simulink model "dspilbc"  (Simulink 8.3)
settings: Solver=FixedStepDiscrete  StartTime=0.0  StopTime=inf  RelTol=1e-3
InitFcn:
  | ilbcDatatype = get_param([bdroot '/Configuration'],'ilbcDialogDatatype');
  | if strcmp(get_param([bdroot '/Configuration'],'ilbcDialogMode'), '13.33 kbit/sec mode')
  |   ilbcMode = 1;
  | else
  |   ilbcMode = 2;
  | end
model workspace: external: MAT-File dspilbcdata.mat (data not in the file)
undefined symbols (not defined in the file or in its folder): dfilt, ilbc, Newton, Raphson
libraries: simulink x36, dspmtrx3 x27, dspsigops x13, dsparch4 x10, dspquant2 x9, dspilbclib x8, dspstat3 x8, dspsrcs4 x2, dspvision x1, dspmisc x1, dspsnks4 x1, dsplp x1
(part 2 of 3)

== system dspilbc/iLBC Encoder/Create Packet (3.8)/Pack Packet ==
  Values : Inport
  Bitwise Operator1 : simulink/Logic and Bit Operations/Bitwise Operator  logicop=AND  UseBitMask=on  BitMask=128  BitMaskRealWorld=Stored Integer
  Bitwise Operator2 : simulink/Logic and Bit Operations/Bitwise Operator  logicop=AND  UseBitMask=on  BitMask=64  BitMaskRealWorld=Stored Integer
  Bitwise Operator3 : simulink/Logic and Bit Operations/Bitwise Operator  logicop=AND  UseBitMask=on  BitMask=32  BitMaskRealWorld=Stored Integer
  Bitwise Operator4 : simulink/Logic and Bit Operations/Bitwise Operator  logicop=AND  UseBitMask=on  BitMask=16  BitMaskRealWorld=Stored Integer
  Bitwise Operator5 : simulink/Logic and Bit Operations/Bitwise Operator  logicop=AND  UseBitMask=on  BitMask=8  BitMaskRealWorld=Stored Integer
  Bitwise Operator6 : simulink/Logic and Bit Operations/Bitwise Operator  logicop=AND  UseBitMask=on  BitMask=4  BitMaskRealWorld=Stored Integer
  Bitwise Operator7 : simulink/Logic and Bit Operations/Bitwise Operator  logicop=AND  UseBitMask=on  BitMask=2  BitMaskRealWorld=Stored Integer
  Bitwise Operator8 : simulink/Logic and Bit Operations/Bitwise Operator  logicop=AND  UseBitMask=on  BitMask=1  BitMaskRealWorld=Stored Integer
  Compare To Constant8 : simulink/Logic and Bit Operations/Compare To Constant  relop=~=  const=0  OutDataTypeStr=boolean  ZeroCross=off
  Constant : Constant  Value=[128 64 32 16 8 4 2 1]'  VectorParams1D=off  OutDataTypeStr=uint8
  Matrix Concatenate : Concatenate  NumInputs=8  Mode=Multidimensional array
  Matrix Multiply : Product  Multiplication=Matrix(*)  OutDataTypeStr=uint8
  Reshape : Reshape  OutputDimensionality=Customize  OutputDimensions=[ilbc.NO_OF_BYTES{ilbcMode} 8]
  Selector : Selector  NumberOfDimensions=2  InputPortWidth=3  IndexOptions=Index vector (dialog),Select all  Indices=ilbc.bit_packTbl{ilbcMode},1  OutputSizes=1,1
  Packet : Outport
  wires:
  Matrix Concatenate/1 -> Compare To Constant8/1
  Values/1 -> Bitwise Operator7/1, Bitwise Operator8/1, Bitwise Operator6/1, Bitwise Operator5/1, Bitwise Operator4/1, Bitwise Operator3/1, Bitwise Operator2/1, Bitwise Operator1/1
  Constant/1 -> Matrix Multiply/2
  Matrix Multiply/1 -> Packet/1
  Reshape/1 -> Matrix Multiply/1
  Selector/1 -> Reshape/1
  Bitwise Operator8/1 -> Matrix Concatenate/8
  Bitwise Operator7/1 -> Matrix Concatenate/7
  Bitwise Operator6/1 -> Matrix Concatenate/6
  Bitwise Operator5/1 -> Matrix Concatenate/5
  Bitwise Operator4/1 -> Matrix Concatenate/4
  Bitwise Operator3/1 -> Matrix Concatenate/3
  Bitwise Operator2/1 -> Matrix Concatenate/2
  Bitwise Operator1/1 -> Matrix Concatenate/1
  Compare To Constant8/1 -> Selector/1

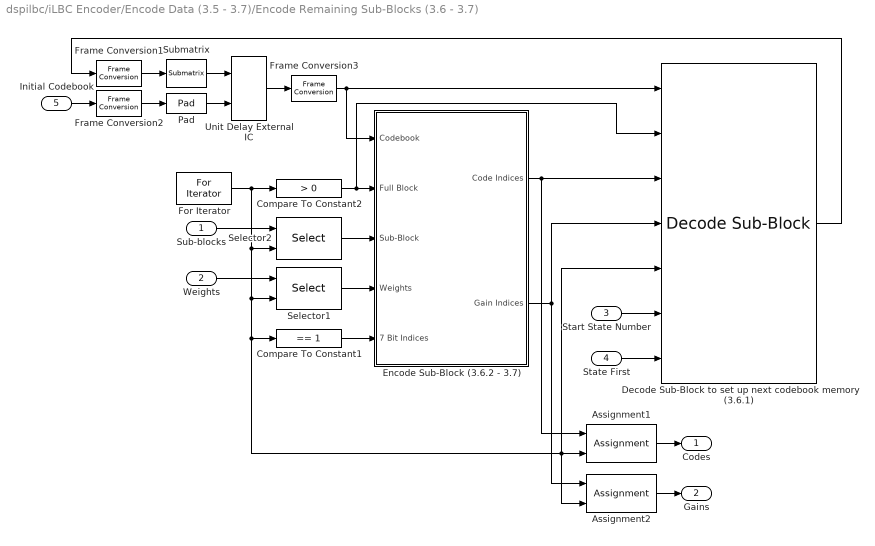
== system dspilbc/iLBC Encoder/Encode Data (3.5 - 3.7)/Encode Remaining Sub-Blocks (3.6 - 3.7) ==
  Sub-blocks : Inport
  Weights : Inport  Port=2
  Start State Number : Inport  Port=3
  State First : Inport  Port=4
  Initial Codebook : Inport  Port=5
  Assignment1 : Assignment  NumberOfDimensions=2  IndexMode=Zero-based  OutputInitialize=Specify size for each dimension in table  IndexOptions=Assign all,Index vector (port)  Indices=1,1  OutputSizes=3,ilbc.NSUB{ilbcMode}-1
  Assignment2 : Assignment  NumberOfDimensions=2  IndexMode=Zero-based  OutputInitialize=Specify size for each dimension in table  IndexOptions=Assign all,Index vector (port)  Indices=1,1  OutputSizes=3,ilbc.NSUB{ilbcMode}-1
  Compare To Constant1 : simulink/Logic and Bit Operations/Compare To Constant  relop===  const=1  OutDataTypeStr=uint8  ZeroCross=off
  Compare To Constant2 : simulink/Logic and Bit Operations/Compare To Constant  relop=>  const=0  OutDataTypeStr=uint8  ZeroCross=off
  Decode Sub-Block to set up next codebook memory (3.6.1) : dspilbclib/Decode Sub-Block
  Encode Sub-Block (3.6.2 - 3.7) : Subsystem  TreatAsAtomicUnit=on
  For Iterator : ForIterator  ResetStates=reset  IterationLimit=ilbc.NSUB{ilbcMode}-1  IndexMode=Zero-based
  Frame Conversion1 : FrameConversion  OutFrame=Sample-based
  Frame Conversion2 : FrameConversion  OutFrame=Sample-based
  Frame Conversion3 : FrameConversion
  Pad : dspsigops/Pad  padAlong=Columns  dimsToPad=1  valSrc=Specify via dialog  padVal=0  spec=Pad size  padNumOutRowsSpecMethod=User-specified  numOutRows=ilbc.BLOCKL{ilbcMode}-40  padNumOutColsSpecMethod=User-specified  numOutCols=1  isVarDimsMode=off  padBeginning=90  padEnd=0  outSizeMode=User-specified  outSize=1  padSigAt=Beginning  trunc_flag=None  roundingMode=Floor  overflowMode=off  truncOrWrapMode=Truncate  wrap_flag=None
  Selector1 : Selector  NumberOfDimensions=2  IndexMode=Zero-based  InputPortWidth=3  IndexOptions=Select all,Index vector (port)  Indices=-1,0
  Selector2 : Selector  NumberOfDimensions=2  IndexMode=Zero-based  InputPortWidth=3  IndexOptions=Select all,Index vector (port)  Indices=-1,0
  Submatrix : dspmtrx3/Submatrix  RowSpan=Range of rows  RowStartMode=Index  RowStartIndex=41  RowEndMode=Last  RowEndIndex=1  ColSpan=All columns  ColStartMode=First  ColStartIndex=1  ColEndMode=Last  ColEndIndex=1
  Unit Delay External IC : simulink/Additional Math & Discrete/Additional Discrete/Unit Delay External IC  tsamp=-1
  Codes : Outport
  Gains : Outport  Port=2
  wires:
  Encode Sub-Block (3.6.2 - 3.7)/2(Gain Indices) -> Assignment2/1, Decode Sub-Block to set up next codebook memory (3.6.1)/4
  Encode Sub-Block (3.6.2 - 3.7)/1(Code Indices) -> Assignment1/1, Decode Sub-Block to set up next codebook memory (3.6.1)/3
  Compare To Constant2/1 -> Encode Sub-Block (3.6.2 - 3.7)/2(Full Block), Decode Sub-Block to set up next codebook memory (3.6.1)/2
  Frame Conversion1/1 -> Submatrix/1
  Decode Sub-Block to set up next codebook memory (3.6.1)/1 -> Frame Conversion1/1
  Frame Conversion2/1 -> Pad/1
  For Iterator/1 -> Compare To Constant2/1, Selector2/2, Assignment2/2, Assignment1/2, Decode Sub-Block to set up next codebook memory (3.6.1)/5, Compare To Constant1/1, Selector1/2
  Frame Conversion3/1 -> Encode Sub-Block (3.6.2 - 3.7)/1(Codebook), Decode Sub-Block to set up next codebook memory (3.6.1)/1
  Assignment2/1 -> Gains/1
  Assignment1/1 -> Codes/1
  Weights/1 -> Selector1/1
  Sub-blocks/1 -> Selector2/1
  Initial Codebook/1 -> Frame Conversion2/1
  Compare To Constant1/1 -> Encode Sub-Block (3.6.2 - 3.7)/5(7 Bit Indices)
  Selector1/1 -> Encode Sub-Block (3.6.2 - 3.7)/4(Weights)
  Selector2/1 -> Encode Sub-Block (3.6.2 - 3.7)/3(Sub-Block)
  Submatrix/1 -> Unit Delay External IC/1
  Pad/1 -> Unit Delay External IC/2
  Unit Delay External IC/1 -> Frame Conversion3/1
  Start State Number/1 -> Decode Sub-Block to set up next codebook memory (3.6.1)/6
  State First/1 -> Decode Sub-Block to set up next codebook memory (3.6.1)/7

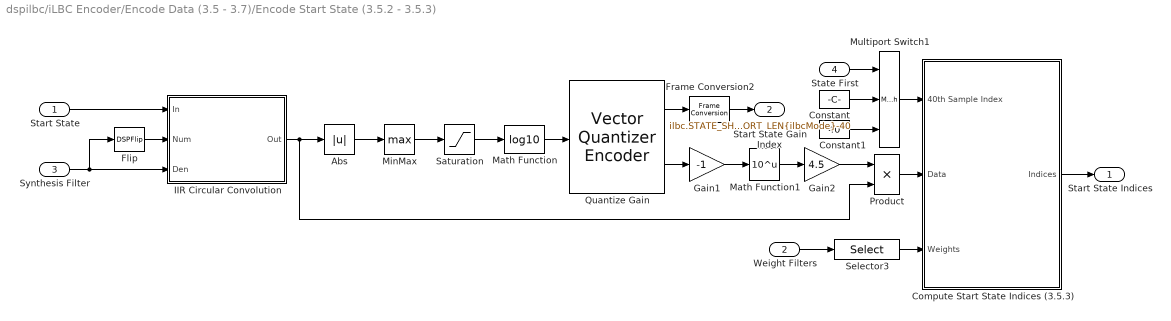
== system dspilbc/iLBC Encoder/Encode Data (3.5 - 3.7)/Encode Start State (3.5.2 - 3.5.3) ==
  Start State : Inport
  Weight Filters : Inport  Port=2
  Synthesis Filter : Inport  Port=3
  State First : Inport  Port=4
  Abs : Abs
  Compute Start State Indices (3.5.3) : Subsystem  TreatAsAtomicUnit=on
  Constant : Constant  Value=ilbc.STATE_SHORT_LEN{ilbcMode}-40  OutDataTypeStr=Inherit: Inherit via back propagation
  Constant1 : Constant  Value=40  OutDataTypeStr=Inherit: Inherit via back propagation
  Flip : DSPFlip
  Frame Conversion2 : FrameConversion  OutFrame=Sample-based
  Gain1 : Gain  Gain=-1  ParamDataTypeStr=Inherit: Same as input
  Gain2 : Gain  Gain=4.5  ParamDataTypeStr=Inherit: Same as input
  IIR Circular Convolution : Subsystem  TreatAsAtomicUnit=on
  Math Function : Math  Operator=log10  SaturateOnIntegerOverflow=on
  Math Function1 : Math  Operator=10^u  SaturateOnIntegerOverflow=on
  MinMax : MinMax  Function=max
  Multiport Switch1 : MultiPortSwitch  DataPortOrder=Zero-based contiguous  Inputs=2  zeroidx=on
  Product : Product  RndMeth=Zero
  Quantize Gain : dspquant2/Vector Quantizer Encoder  CBsource=Specify via dialog  codebook=ilbc.state_frgqTbl  distMeasure=Squared error  wgtSrc=Input port  weights=[1 1 1]  tieBreakRule=Choose the lower index  outQU=on  outQError=off  idtype=uint8  roundingMode=Floor  overflowMode=off
      settings: additionalParams=on
  Saturation : Saturate  UpperLimit=inf  LowerLimit=10
  Selector3 : Selector  NumberOfDimensions=2  InputPortWidth=3  IndexOptions=Index vector (dialog),Select all  Indices=2:11,-1
  Start State Indices : Outport
  Start State Gain Index : Outport  Port=2
  wires:
  Gain2/1 -> Product/1
  Product/1 -> Compute Start State Indices (3.5.3)/2(Data)
  Weight Filters/1 -> Selector3/1
  Multiport Switch1/1 -> Compute Start State Indices (3.5.3)/1(40th Sample Index)
  State First/1 -> Multiport Switch1/1
  Gain1/1 -> Math Function1/1
  IIR Circular Convolution/1(Out) -> Product/2, Abs/1
  Constant1/1 -> Multiport Switch1/3
  Constant/1 -> Multiport Switch1/2
  Selector3/1 -> Compute Start State Indices (3.5.3)/3(Weights)
  Math Function/1 -> Quantize Gain/1
  Math Function1/1 -> Gain2/1
  Frame Conversion2/1 -> Start State Gain Index/1
  Compute Start State Indices (3.5.3)/1(Indices) -> Start State Indices/1
  Start State/1 -> IIR Circular Convolution/1(In)
  Saturation/1 -> Math Function/1
  Synthesis Filter/1 -> IIR Circular Convolution/3(Den), Flip/1
  Quantize Gain/1 -> Frame Conversion2/1
  Quantize Gain/2 -> Gain1/1
  MinMax/1 -> Saturation/1
  Abs/1 -> MinMax/1
  Flip/1 -> IIR Circular Convolution/2(Num)

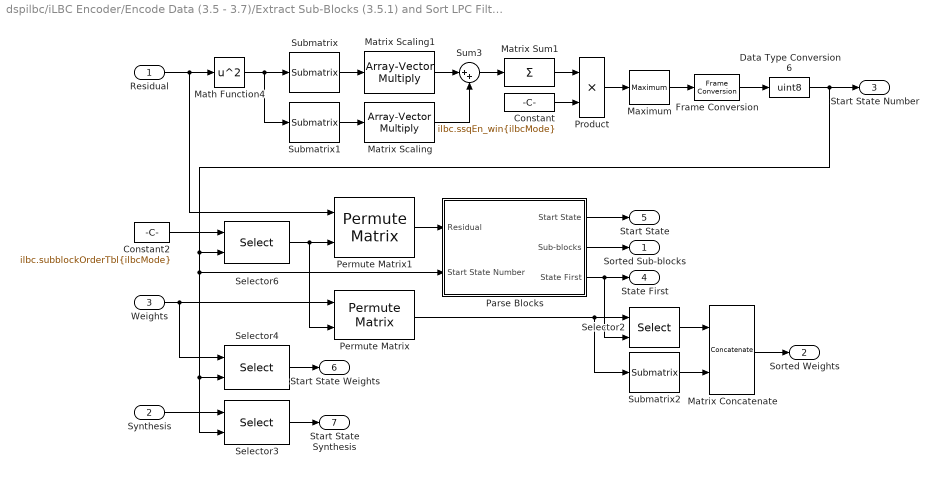
== system dspilbc/iLBC Encoder/Encode Data (3.5 - 3.7)/Extract Sub-Blocks (3.5.1) and Sort LPC Filters ==
  Residual : Inport
  Synthesis : Inport  Port=2
  Weights : Inport  Port=3
  Constant : Constant  Value=ilbc.ssqEn_win{ilbcMode}  VectorParams1D=off  OutDataTypeStr=Inherit: Inherit via back propagation
      settings: SamplingMode=Frame based
  Constant2 : Constant  Value=ilbc.subblockOrderTbl{ilbcMode}  OutDataTypeStr=uint8
  Data Type Conversion6 : DataTypeConversion  OutDataTypeStr=uint8
  Frame Conversion : FrameConversion  OutFrame=Sample-based
  Math Function4 : Math  Operator=square  SaturateOnIntegerOverflow=on
  Matrix Concatenate : Concatenate  Mode=Multidimensional array  ConcatenateDimension=2
  Matrix Scaling : dspmtrx3/Array-Vector Multiply  mode=Mute  saveAsFlag=0  Dimension=1  V_Source=Dialog parameter  V_VectFromMask=ilbc.sampEn_win2  firstCoeffSignedness=Auto  firstCoeffDataTypeStr=Inherit: Same word length as input  firstCoeffLastDataTypeStr=Inherit: Same word length as input  firstCoeffMin=[]  firstCoeffMax=[]  outputSignedness=Auto  outputMin=[]  outputMax=[]  accumSignedness=Auto  prodOutputSignedness=Auto  roundingMode=Floor  overflowMode=off
  Matrix Scaling1 : dspmtrx3/Array-Vector Multiply  mode=Mute  saveAsFlag=0  Dimension=1  V_Source=Dialog parameter  V_VectFromMask=ilbc.sampEn_win1  firstCoeffSignedness=Auto  firstCoeffDataTypeStr=Inherit: Same word length as input  firstCoeffLastDataTypeStr=Inherit: Same word length as input  firstCoeffMin=[]  firstCoeffMax=[]  outputSignedness=Auto  outputMin=[]  outputMax=[]  accumSignedness=Auto  prodOutputSignedness=Auto  roundingMode=Floor  overflowMode=off
  Matrix Sum1 : Sum  Inputs=+  CollapseMode=Specified dimension  OutDataTypeStr=Inherit: Same as accumulator
  Maximum : dspstat3/Maximum  fcn=Index  reset=None  InputProcessing=Columns as channels (frame based)  indexBase=One  operateOver=Each row  Dimension=1  colComp=on  operation=maximum  roiEnable=off  roiType=Rectangles  roiPortion=Entire ROI  roiOutput=Individual statistics for each ROI  roiFlag=off  accumDataTypeStr=Inherit: Same as product output  accumLastDataTypeStr=Inherit: Same as product output  roundingMode=Floor  overflowMode=off
  Parse Blocks : Subsystem
  Permute Matrix : dspmtrx3/Permute Matrix  mode=Columns  ZeroOneIdxMode=One-based  errmode=Clip index  checkDims=off
  Permute Matrix1 : dspmtrx3/Permute Matrix  mode=Columns  ZeroOneIdxMode=One-based  errmode=Clip index  checkDims=off
  Product : Product  RndMeth=Zero
  Selector2 : Selector  NumberOfDimensions=2  IndexMode=Zero-based  InputPortWidth=3  IndexOptions=Select all,Index vector (port)  Indices=-1,1:2
  Selector3 : Selector  NumberOfDimensions=2  InputPortWidth=3  IndexOptions=Select all,Index vector (port)  Indices=-1,-1  OutputSizes=2,2
  Selector4 : Selector  NumberOfDimensions=2  InputPortWidth=3  IndexOptions=Select all,Starting index (port)  Indices=-1,-1  OutputSizes=2,2
  Selector6 : Selector  NumberOfDimensions=2  InputPortWidth=3  IndexOptions=Index vector (port),Select all  Indices=-1,-1
  Submatrix : dspmtrx3/Submatrix  RowSpan=All rows  RowStartMode=First  RowStartIndex=1  RowEndMode=Last  RowEndIndex=1  ColSpan=Range of columns  ColStartMode=First  ColStartIndex=1  ColEndMode=Offset from last  ColEndIndex=1
  Submatrix1 : dspmtrx3/Submatrix  RowSpan=All rows  RowStartMode=First  RowStartIndex=1  RowEndMode=Last  RowEndIndex=1  ColSpan=Range of columns  ColStartMode=Index  ColStartIndex=2  ColEndMode=Last  ColEndIndex=1
  Submatrix2 : dspmtrx3/Submatrix  RowSpan=All rows  RowStartMode=Index  RowStartIndex=1  RowEndMode=Last  RowEndIndex=1  ColSpan=Range of columns  ColStartMode=Index  ColStartIndex=3  ColEndMode=Last  ColEndIndex=1
  Sum3 : Sum  Inputs=|++
  Sorted Sub-blocks : Outport
  Sorted Weights : Outport  Port=2
  Start State Number : Outport  Port=3
  State First : Outport  Port=4
  Start State : Outport  Port=5
  Start State Weights : Outport  Port=6
  Start State Synthesis : Outport  Port=7
  wires:
  Permute Matrix1/1 -> Parse Blocks/1(Residual)
  Selector6/1 -> Permute Matrix/2, Permute Matrix1/2
  Constant2/1 -> Selector6/1
  Data Type Conversion6/1 -> Selector6/2, Selector3/2, Selector4/2, Parse Blocks/2(Start State Number), Start State Number/1
  Matrix Concatenate/1 -> Sorted Weights/1
  Submatrix2/1 -> Matrix Concatenate/2
  Selector2/1 -> Matrix Concatenate/1
  Permute Matrix/1 -> Submatrix2/1, Selector2/1
  Selector4/1 -> Start State Weights/1
  Weights/1 -> Selector4/1, Permute Matrix/1
  Synthesis/1 -> Selector3/1
  Selector3/1 -> Start State Synthesis/1
  Frame Conversion/1 -> Data Type Conversion6/1
  Product/1 -> Maximum/1
  Constant/1 -> Product/2
  Matrix Sum1/1 -> Product/1
  Sum3/1 -> Matrix Sum1/1
  Matrix Scaling/1 -> Sum3/2
  Matrix Scaling1/1 -> Sum3/1
  Submatrix1/1 -> Matrix Scaling/1
  Submatrix/1 -> Matrix Scaling1/1
  Math Function4/1 -> Submatrix1/1, Submatrix/1
  Residual/1 -> Permute Matrix1/1, Math Function4/1
  Parse Blocks/2(Sub-blocks) -> Sorted Sub-blocks/1
  Parse Blocks/1(Start State) -> Start State/1
  Parse Blocks/3(State First) -> Selector2/2, State First/1
  Maximum/1 -> Frame Conversion/1

== system dspilbc/iLBC Encoder/Encoder LPC Analysis (3.2)/LSF Quantization (3.2.4) ==
  LSF Vectors : Inport
  Concatenation of Quantized LSFs : Concatenate  NumInputs=3  Mode=Multidimensional array
  Concatenation of Quantized LSFs1 : Concatenate  NumInputs=3  Mode=Multidimensional array
  Frame Conversion1 : FrameConversion  OutFrame=Sample-based
  Reshape : Reshape  OutputDimensionality=Column vector (2-D)
  Saturation : Saturate  UpperLimit=3.14  LowerLimit=0.01
  Selector1 : Selector  NumberOfDimensions=2  InputPortWidth=3  IndexOptions=Index vector (dialog),Select all  Indices=1:3,-1
  Selector2 : Selector  NumberOfDimensions=2  InputPortWidth=3  IndexOptions=Index vector (dialog),Select all  Indices=4:6,-1
  Selector3 : Selector  NumberOfDimensions=2  InputPortWidth=3  IndexOptions=Index vector (dialog),Select all  Indices=7:10,-1
  Sort : dspstat3/Sort  otype=Value  dir=Ascending  sortAlg=Quick sort  roundingMode=Floor  overflowMode=off
  VQ of LSF: 1st subvector : dspquant2/Vector Quantizer Encoder  CBsource=Specify via dialog  codebook=ilbc.lsfCbTbl1  distMeasure=Squared error  wgtSrc=Input port  weights=[1 1 1]  tieBreakRule=Choose the lower index  outQU=on  outQError=off  idtype=uint8  roundingMode=Floor  overflowMode=off
      settings: additionalParams=on
  VQ of LSF: 2nd subvector : dspquant2/Vector Quantizer Encoder  CBsource=Specify via dialog  codebook=ilbc.lsfCbTbl2  distMeasure=Squared error  wgtSrc=Input port  weights=[1 1 1]  tieBreakRule=Choose the lower index  outQU=on  outQError=off  idtype=uint8  roundingMode=Floor  overflowMode=off
      settings: additionalParams=on
  VQ of LSF: 3rd subvector : dspquant2/Vector Quantizer Encoder  CBsource=Specify via dialog  codebook=ilbc.lsfCbTbl3  distMeasure=Squared error  wgtSrc=Input port  weights=[1 1 1]  tieBreakRule=Choose the lower index  outQU=on  outQError=off  idtype=uint8  roundingMode=Floor  overflowMode=off
      settings: additionalParams=on
  LSF Indices : Outport
  Quantized LSF Vectors : Outport  Port=2
  wires:
  Reshape/1 -> Frame Conversion1/1
  Selector3/1 -> VQ of LSF: 3rd subvector/1
  Selector2/1 -> VQ of LSF: 2nd subvector/1
  Selector1/1 -> VQ of LSF: 1st subvector/1
  Frame Conversion1/1 -> LSF Indices/1
  VQ of LSF: 3rd subvector/1 -> Concatenation of Quantized LSFs1/3
  VQ of LSF: 2nd subvector/1 -> Concatenation of Quantized LSFs1/2
  VQ of LSF: 1st subvector/1 -> Concatenation of Quantized LSFs1/1
  Concatenation of Quantized LSFs1/1 -> Reshape/1
  Saturation/1 -> Quantized LSF Vectors/1
  LSF Vectors/1 -> Selector2/1, Selector3/1, Selector1/1
  Sort/1 -> Saturation/1
  VQ of LSF: 3rd subvector/2 -> Concatenation of Quantized LSFs/3
  Concatenation of Quantized LSFs/1 -> Sort/1
  VQ of LSF: 2nd subvector/2 -> Concatenation of Quantized LSFs/2
  VQ of LSF: 1st subvector/2 -> Concatenation of Quantized LSFs/1

== system dspilbc/iLBC Encoder/Encode Data (3.5 - 3.7)/Encode Remaining Sub-Blocks (3.6 - 3.7)/Encode Sub-Block (3.6.2 - 3.7) ==
  Codebook : Inport
  Full Block : Inport  Port=2
  Sub-Block : Inport  Port=3
  Weights : Inport  Port=4
  7 Bit Indices : Inport  Port=5
  3 Stage Sub-Block Encoder (3.6.4) : Subsystem  TreatAsAtomicUnit=on
  Adjust First Gain Index (3.7) : Subsystem  TreatAsAtomicUnit=on
  Compute Codebooks (3.6.2 - 3.6.3) : Subsystem
  Code Indices : Outport
  Gain Indices : Outport  Port=2
  wires:
  Codebook/1 -> Compute Codebooks (3.6.2 - 3.6.3)/1(Codebook)
  3 Stage Sub-Block Encoder (3.6.4)/4(Quantized Gain) -> Adjust First Gain Index (3.7)/4(Quantized Gain)
  3 Stage Sub-Block Encoder (3.6.4)/3(Quantized Target) -> Adjust First Gain Index (3.7)/3(Quantized Target)
  3 Stage Sub-Block Encoder (3.6.4)/2(Gain Indices) -> Adjust First Gain Index (3.7)/2(Gain Indices)
  3 Stage Sub-Block Encoder (3.6.4)/1(Code Indices) -> Code Indices/1
  Adjust First Gain Index (3.7)/1(Adjusted Gain Indices) -> Gain Indices/1
  Sub-Block/1 -> Compute Codebooks (3.6.2 - 3.6.3)/2(Sub-Block)
  Weights/1 -> Compute Codebooks (3.6.2 - 3.6.3)/3(Weights)
  Compute Codebooks (3.6.2 - 3.6.3)/1(Target) -> 3 Stage Sub-Block Encoder (3.6.4)/1(Target), Adjust First Gain Index (3.7)/1(Target)
  Compute Codebooks (3.6.2 - 3.6.3)/2(Codebooks) -> 3 Stage Sub-Block Encoder (3.6.4)/2(Codebooks)
  Compute Codebooks (3.6.2 - 3.6.3)/3(Augmented) -> 3 Stage Sub-Block Encoder (3.6.4)/3(Augmented)
  Compute Codebooks (3.6.2 - 3.6.3)/4(Norms) -> 3 Stage Sub-Block Encoder (3.6.4)/4("Norms ")
  Full Block/1 -> Compute Codebooks (3.6.2 - 3.6.3)/4(Full Block), 3 Stage Sub-Block Encoder (3.6.4)/6(Full Block)
  7 Bit Indices/1 -> 3 Stage Sub-Block Encoder (3.6.4)/5(7 Bit Indices)

== system dspilbc/iLBC Encoder/Encode Data (3.5 - 3.7)/Encode Start State (3.5.2 - 3.5.3)/Compute Start State Indices (3.5.3) ==
  40th Sample Index : Inport
  Data : Inport  Port=2
  Weights : Inport  Port=3
  Assignment : Assignment  NumberOfDimensions=2  OutputInitialize=Specify size for each dimension in table  IndexOptions=Index vector (port),Assign all  Indices=1,-1  OutputSizes=ilbc.STATE_SHORT_LEN{ilbcMode},1
  Delay : dspsigops/Delay  dly_unit=Samples  delay=1  ic_detail=off  dif_ic_for_ch=off  dif_ic_for_dly=off  ic=0  reset_popup=None
  Delay1 : dspsigops/Delay  dly_unit=Samples  delay=1  ic_detail=off  dif_ic_for_ch=off  dif_ic_for_dly=off  ic=0  reset_popup=None
  Dot Product : DotProduct  InputSameDT=on  OutDataTypeStr=Inherit: Inherit via internal rule
  Dot Product1 : DotProduct  InputSameDT=on  OutDataTypeStr=Inherit: Inherit via internal rule
  For Iterator : ForIterator  ResetStates=reset  IterationLimit=ilbc.STATE_SHORT_LEN{ilbcMode}
  Frame Conversion1 : FrameConversion  OutFrame=Sample-based
  Relational Operator : RelationalOperator  Operator=>  OutDataTypeStr=uint(8)
  Selector1 : Selector  NumberOfDimensions=2  IndexMode=Zero-based  InputPortWidth=3  IndexOptions=Select all,Index vector (port)  Indices=-1,-1
  Selector2 : Selector  NumberOfDimensions=2  InputPortWidth=3  IndexOptions=Index vector (port),Select all  Indices=-1,-1
  Sum : Sum  Inputs=+|+  OutDataTypeStr=Inherit: Inherit via back propagation
  Sum1 : Sum  Inputs=+-|
  Sum2 : Sum  Inputs=|-+
  Tapped Delay : simulink/Discrete/Tapped Delay  vinit=0.0  samptime=-1  NumDelays=9  DelayOrder=Newest  includeCurrent=on
  Tapped Delay1 : simulink/Discrete/Tapped Delay  vinit=0.0  samptime=-1  NumDelays=9  DelayOrder=Newest  includeCurrent=on
  Vector Quantizer Encoder : dspquant2/Vector Quantizer Encoder  CBsource=Specify via dialog  codebook=ilbc.state_sq3Tbl  distMeasure=Squared error  wgtSrc=Specify via dialog  weights=[1 1 1]  tieBreakRule=Choose the lower index  outQU=on  outQError=off  idtype=uint8  roundingMode=Floor  overflowMode=on
      settings: additionalParams=on
  Indices : Outport
  wires:
  For Iterator/1 -> Assignment/2, Selector2/2, Relational Operator/1
  Dot Product1/1 -> Sum2/1
  Delay1/1 -> Dot Product1/1
  Selector2/1 -> Sum2/2
  Sum2/1 -> Sum/1, Tapped Delay1/1
  Tapped Delay1/1 -> Delay1/1
  Sum1/1 -> Tapped Delay/1
  Tapped Delay/1 -> Delay/1
  Delay/1 -> Dot Product/2
  Dot Product/1 -> Sum1/2, Sum/2
  Selector1/1 -> Dot Product1/2, Dot Product/1
  Relational Operator/1 -> Selector1/2
  Weights/1 -> Selector1/1
  Data/1 -> Frame Conversion1/1
  Vector Quantizer Encoder/2 -> Sum1/1
  Vector Quantizer Encoder/1 -> Assignment/1
  Sum/1 -> Vector Quantizer Encoder/1
  40th Sample Index/1 -> Relational Operator/2
  Assignment/1 -> Indices/1
  Frame Conversion1/1 -> Selector2/1

== system dspilbc/iLBC Encoder/Encode Data (3.5 - 3.7)/Encode Start State (3.5.2 - 3.5.3)/IIR Circular Convolution ==
  In : Inport
  Num : Inport  Port=2
  Den : Inport  Port=3
  Digital Filter : dsparch4/Digital Filter  TypePopup=IIR (poles & zeros)  IIRFiltStruct=Direct form II transposed  AllPoleFiltStruct=Direct form  FIRFiltStruct=Direct form  CoeffSource=Input port(s)  NumCoeffs=[1 2]  DenCoeffs=[1 0.1]  BiQuadCoeffs=[1 0.3 0.4 1 0.1 0.2]  LatticeCoeffs=[0.2 0.4]  denIgnore=on  FiltPerSampPopup=One filter per frame  IC=0  ICnum=0  ICden=0  roundingMode=Floor  overflowMode=off  ScaleValues=1  scaleValueFracLength=14  stageInFracLength=15  stageOutFracLength=15  FilterSource=Input port(s)  dfiltObjectName=dfilt.dffir([1 2 1])  InputProcessing=Columns as channels (frame based)
  For Iterator : ForIterator  ResetStates=reset  IterationLimit=2  ShowIterationPort=off
  Out : Outport
  wires:
  Den/1 -> Digital Filter/3
  Num/1 -> Digital Filter/2
  In/1 -> Digital Filter/1
  Digital Filter/1 -> Out/1

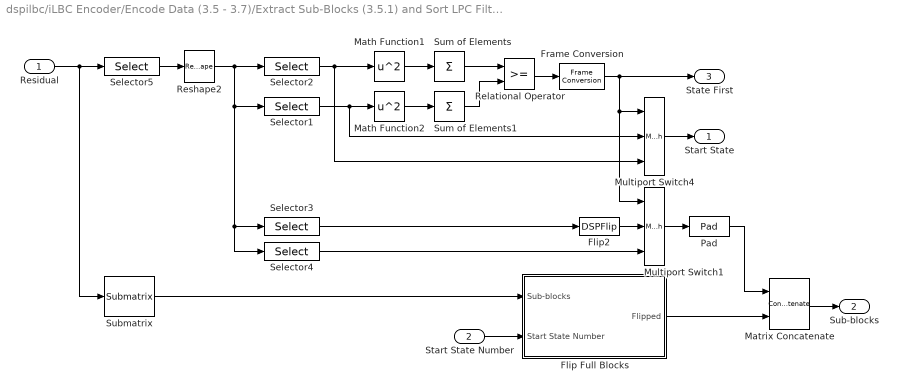
== system dspilbc/iLBC Encoder/Encode Data (3.5 - 3.7)/Extract Sub-Blocks (3.5.1) and Sort LPC Filters/Parse Blocks ==
  Residual : Inport
  Start State Number : Inport  Port=2
  Flip Full Blocks : Subsystem  TreatAsAtomicUnit=on
  Flip2 : DSPFlip
  Frame Conversion : FrameConversion  OutFrame=Sample-based
  Math Function1 : Math  Operator=square  SaturateOnIntegerOverflow=on
  Math Function2 : Math  Operator=square  SaturateOnIntegerOverflow=on
  Matrix Concatenate : Concatenate  Mode=Multidimensional array  ConcatenateDimension=2
  Multiport Switch1 : MultiPortSwitch  DataPortOrder=Zero-based contiguous  Inputs=2  zeroidx=on
  Multiport Switch4 : MultiPortSwitch  DataPortOrder=Zero-based contiguous  Inputs=2  zeroidx=on
  Pad : dspsigops/Pad  padAlong=Columns  dimsToPad=1  valSrc=Specify via dialog  padVal=0  spec=Output size  padNumOutRowsSpecMethod=User-specified  numOutRows=40  padNumOutColsSpecMethod=User-specified  numOutCols=1  isVarDimsMode=off  padBeginning=0  padEnd=0  outSizeMode=User-specified  outSize=1  padSigAt=End  trunc_flag=None  roundingMode=Floor  overflowMode=off  truncOrWrapMode=Truncate  wrap_flag=None
  Relational Operator : RelationalOperator  OutDataTypeStr=uint(8)
  Reshape2 : Reshape  OutputDimensionality=Column vector (2-D)
  Selector1 : Selector  NumberOfDimensions=2  InputPortWidth=3  IndexOptions=Index vector (dialog),Select all  Indices=(80-ilbc.STATE_SHORT_LEN{ilbcMode}+1):80,-1
  Selector2 : Selector  NumberOfDimensions=2  InputPortWidth=3  IndexOptions=Index vector (dialog),Select all  Indices=1:ilbc.STATE_SHORT_LEN{ilbcMode},-1
  Selector3 : Selector  NumberOfDimensions=2  InputPortWidth=3  IndexOptions=Starting index (dialog),Select all  Indices=1,-1  OutputSizes=80-ilbc.STATE_SHORT_LEN{ilbcMode},1
  Selector4 : Selector  NumberOfDimensions=2  InputPortWidth=3  IndexOptions=Index vector (dialog),Select all  Indices=(ilbc.STATE_SHORT_LEN{ilbcMode}+1):80,-1
  Selector5 : Selector  NumberOfDimensions=2  InputPortWidth=3  IndexOptions=Select all,Index vector (dialog)  Indices=1:ilbc.STATE_SHORT_LEN{ilbcMode},1:2
  Submatrix : dspmtrx3/Submatrix  RowSpan=All rows  RowStartMode=First  RowStartIndex=1  RowEndMode=Last  RowEndIndex=1  ColSpan=Range of columns  ColStartMode=Index  ColStartIndex=3  ColEndMode=Last  ColEndIndex=1
  Sum of Elements : Sum  Inputs=+
  Sum of Elements1 : Sum  Inputs=+
  Start State : Outport
  Sub-blocks : Outport  Port=2
  State First : Outport  Port=3
  wires:
  Start State Number/1 -> Flip Full Blocks/2(Start State Number)
  Flip2/1 -> Multiport Switch1/2
  Flip Full Blocks/1(Flipped) -> Matrix Concatenate/2
  Submatrix/1 -> Flip Full Blocks/1(Sub-blocks)
  Matrix Concatenate/1 -> Sub-blocks/1
  Pad/1 -> Matrix Concatenate/1
  Multiport Switch1/1 -> Pad/1
  Reshape2/1 -> Selector3/1, Selector4/1, Selector1/1, Selector2/1
  Multiport Switch4/1 -> Start State/1
  Selector5/1 -> Reshape2/1
  Residual/1 -> Selector5/1, Submatrix/1
  Math Function2/1 -> Sum of Elements1/1
  Math Function1/1 -> Sum of Elements/1
  Sum of Elements1/1 -> Relational Operator/2
  Relational Operator/1 -> Frame Conversion/1
  Frame Conversion/1 -> State First/1, Multiport Switch1/1, Multiport Switch4/1
  Sum of Elements/1 -> Relational Operator/1
  Selector3/1 -> Flip2/1
  Selector4/1 -> Multiport Switch1/3
  Selector1/1 -> Math Function2/1, Multiport Switch4/2
  Selector2/1 -> Multiport Switch4/3, Math Function1/1

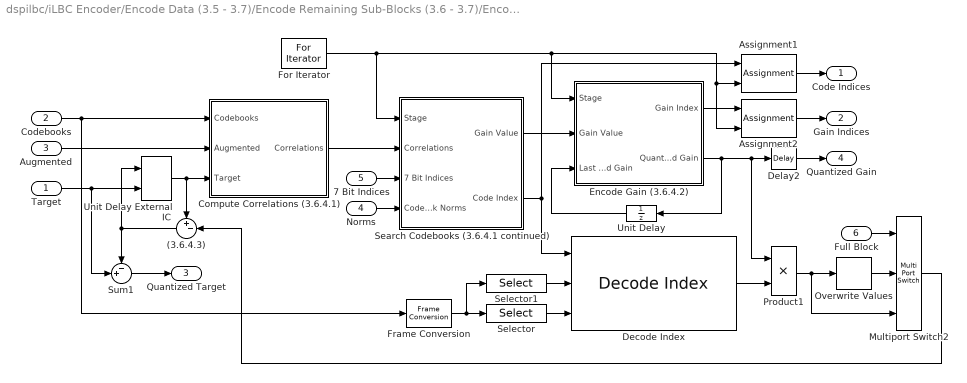
== system dspilbc/iLBC Encoder/Encode Data (3.5 - 3.7)/Encode Remaining Sub-Blocks (3.6 - 3.7)/Encode Sub-Block (3.6.2 - 3.7)/3 Stage Sub-Block Encoder (3.6.4) ==
  Target : Inport
  Codebooks : Inport  Port=2
  Augmented : Inport  Port=3
  "Norms " : Inport  Port=4
  7 Bit Indices : Inport  Port=5
  Full Block : Inport  Port=6
  (3.6.4.3) : Sum  Inputs=+-|
  Assignment1 : Assignment  NumberOfDimensions=2  IndexMode=Zero-based  OutputInitialize=Specify size for each dimension in table  IndexOptions=Index vector (port),Index vector (dialog)  Indices=1,0  OutputSizes=3,1
  Assignment2 : Assignment  NumberOfDimensions=2  IndexMode=Zero-based  OutputInitialize=Specify size for each dimension in table  IndexOptions=Index vector (port),Index vector (dialog)  Indices=1,0  OutputSizes=3,1
  Compute Correlations (3.6.4.1) : Subsystem  TreatAsAtomicUnit=on
  Decode Index : dspilbclib/Decode Index
  Delay2 : dspsigops/Delay  dly_unit=Samples  delay=2  ic_detail=off  dif_ic_for_ch=off  dif_ic_for_dly=off  ic=0  reset_popup=None
  Encode Gain (3.6.4.2) : Subsystem  TreatAsAtomicUnit=on
  For Iterator : ForIterator  ResetStates=reset  IterationLimit=3  IndexMode=Zero-based  IterationVariableDataType=int8
  Frame Conversion : FrameConversion  OutFrame=Sample-based
  Multiport Switch2 : MultiPortSwitch  DataPortOrder=Zero-based contiguous  Inputs=2  zeroidx=on
  Overwrite Values : dspmtrx3/Overwrite Values  OverWriteDiag=Submatrix  valFrom2ndIP=Specify via dialog  ConstValue=0  RowSpan=Range of rows  RowStartMode=First  RowStartIndex=1  RowEndMode=Offset from last  RowEndIndex=80-ilbc.STATE_SHORT_LEN{ilbcMode}  ColSpan=All columns  ColStartMode=First  ColStartIndex=1  ColEndMode=Last  ColEndIndex=1  DiagSpan=Range of elements  DiagStartMode=Index  DiagStartIndex=2  DiagEndMode=Index  DiagEndIndex=4
  Product1 : Product  RndMeth=Zero
  Search Codebooks (3.6.4.1 continued) : Subsystem  TreatAsAtomicUnit=on
  Selector : Selector  NumberOfDimensions=2  InputPortWidth=3  IndexOptions=Select all,Index vector (dialog)  Indices=[1 3],2  OutputSizes=1,1
  Selector1 : Selector  NumberOfDimensions=2  InputPortWidth=3  IndexOptions=Select all,Index vector (dialog)  Indices=[1 3],1  OutputSizes=1,1
  Sum1 : Sum  Inputs=-+|
  Unit Delay : UnitDelay  InitialCondition=1  SampleTime=-1
  Unit Delay External IC : simulink/Additional Math & Discrete/Additional Discrete/Unit Delay External IC  tsamp=-1
  Code Indices : Outport
  Gain Indices : Outport  Port=2
  Quantized Target : Outport  Port=3
  Quantized Gain : Outport  Port=4
  wires:
  Multiport Switch2/1 -> (3.6.4.3)/2
  Product1/1 -> Multiport Switch2/3, Overwrite Values/1
  Frame Conversion/1 -> Selector1/1, Selector/1
  Selector/1 -> Decode Index/3
  Selector1/1 -> Decode Index/2
  Full Block/1 -> Multiport Switch2/1
  Overwrite Values/1 -> Multiport Switch2/2
  Unit Delay External IC/1 -> Compute Correlations (3.6.4.1)/3(Target), (3.6.4.3)/1
  Encode Gain (3.6.4.2)/1(Gain Index) -> Assignment2/1
  Encode Gain (3.6.4.2)/2(Quantized Gain) -> Product1/1, Delay2/1, Unit Delay/1
  Search Codebooks (3.6.4.1 continued)/1(Gain Value) -> Encode Gain (3.6.4.2)/2(Gain Value)
  "Norms "/1 -> Search Codebooks (3.6.4.1 continued)/4(Codebook Norms)
  7 Bit Indices/1 -> Search Codebooks (3.6.4.1 continued)/3(7 Bit Indices)
  (3.6.4.3)/1 -> Sum1/1, Unit Delay External IC/1
  For Iterator/1 -> Assignment1/2, Assignment2/2, Encode Gain (3.6.4.2)/1(Stage), Search Codebooks (3.6.4.1 continued)/1(Stage)
  Assignment2/1 -> Gain Indices/1
  Assignment1/1 -> Code Indices/1
  Decode Index/1 -> Product1/2
  Target/1 -> Sum1/2, Unit Delay External IC/2
  Delay2/1 -> Quantized Gain/1
  Codebooks/1 -> Frame Conversion/1, Compute Correlations (3.6.4.1)/1(Codebooks)
  Search Codebooks (3.6.4.1 continued)/2(Code Index) -> Decode Index/1, Assignment1/1
  Compute Correlations (3.6.4.1)/1(Correlations) -> Search Codebooks (3.6.4.1 continued)/2(Correlations)
  Augmented/1 -> Compute Correlations (3.6.4.1)/2(Augmented)
  Unit Delay/1 -> Encode Gain (3.6.4.2)/3(Last Quantized Gain)
  Sum1/1 -> Quantized Target/1

== system dspilbc/iLBC Encoder/Encode Data (3.5 - 3.7)/Encode Remaining Sub-Blocks (3.6 - 3.7)/Encode Sub-Block (3.6.2 - 3.7)/Adjust First Gain Index (3.7) ==
  Target : Inport
  Gain Indices : Inport  Port=2
  Quantized Target : Inport  Port=3
  Quantized Gain : Inport  Port=4
  Constant : Constant  Value=ilbc.gain_sq5Tbl  VectorParams1D=off  OutDataTypeStr=Inherit: Inherit via back propagation
  Dot Product : DotProduct  InputSameDT=on  OutDataTypeStr=Inherit: Inherit via internal rule
  Dot Product1 : DotProduct  InputSameDT=on  OutDataTypeStr=Inherit: Inherit via internal rule
  Gain : Gain  Gain=2
  Gain1 : Gain  Gain=1:32  OutDataTypeStr=Inherit: Inherit via back propagation
  Logical Operator : Logic  AllPortsSameDT=off  OutDataTypeStr=uint(8)
  Math Function : Math  Operator=square  SaturateOnIntegerOverflow=on
  Math Function1 : Math  Operator=square  SaturateOnIntegerOverflow=on
  Matrix Concatenate : Concatenate  Mode=Multidimensional array
  Maximum1 : dspstat3/Maximum  fcn=Index  reset=None  InputProcessing=Columns as channels (frame based)  indexBase=Zero  operateOver=Each row  Dimension=1  colComp=on  operation=maximum  roiEnable=off  roiType=Rectangles  roiPortion=Entire ROI  roiOutput=Individual statistics for each ROI  roiFlag=off  accumDataTypeStr=Inherit: Same as product output  accumLastDataTypeStr=Inherit: Same as product output  roundingMode=Floor  overflowMode=off
  MinMax : MinMax  Function=max  Inputs=2  OutDataTypeStr=Inherit: Inherit via back propagation
  Product : Product  RndMeth=Zero
  Product1 : Product  RndMeth=Zero
  Relational Operator : RelationalOperator  Operator=>  OutDataTypeStr=uint(8)
  Relational Operator1 : RelationalOperator  Operator=<  OutDataTypeStr=uint(8)
  Selector1 : Selector  NumberOfDimensions=2  InputPortWidth=151  IndexOptions=Index vector (dialog),Select all  Indices=1,1  OutputSizes=1,1
  Selector2 : Selector  NumberOfDimensions=2  InputPortWidth=151  IndexOptions=Index vector (dialog),Select all  Indices=2:3,1  OutputSizes=1,1
  Adjusted Gain Indices : Outport
  wires:
  Gain Indices/1 -> Selector1/1, Selector2/1
  Selector2/1 -> Matrix Concatenate/2
  Selector1/1 -> MinMax/2
  Maximum1/1 -> MinMax/1
  MinMax/1 -> Matrix Concatenate/1
  Matrix Concatenate/1 -> Adjusted Gain Indices/1
  Constant/1 -> Math Function/1, Relational Operator1/1
  Math Function/1 -> Product/2
  Dot Product/1 -> Product/1
  Math Function1/1 -> Product1/1
  Dot Product1/1 -> Product1/2
  Quantized Gain/1 -> Math Function1/1, Gain/1
  Quantized Target/1 -> Dot Product/2, Dot Product/1
  Target/1 -> Dot Product1/2, Dot Product1/1
  Product1/1 -> Relational Operator/1
  Product/1 -> Relational Operator/2
  Gain/1 -> Relational Operator1/2
  Relational Operator/1 -> Logical Operator/1
  Relational Operator1/1 -> Logical Operator/2
  Logical Operator/1 -> Gain1/1
  Gain1/1 -> Maximum1/1

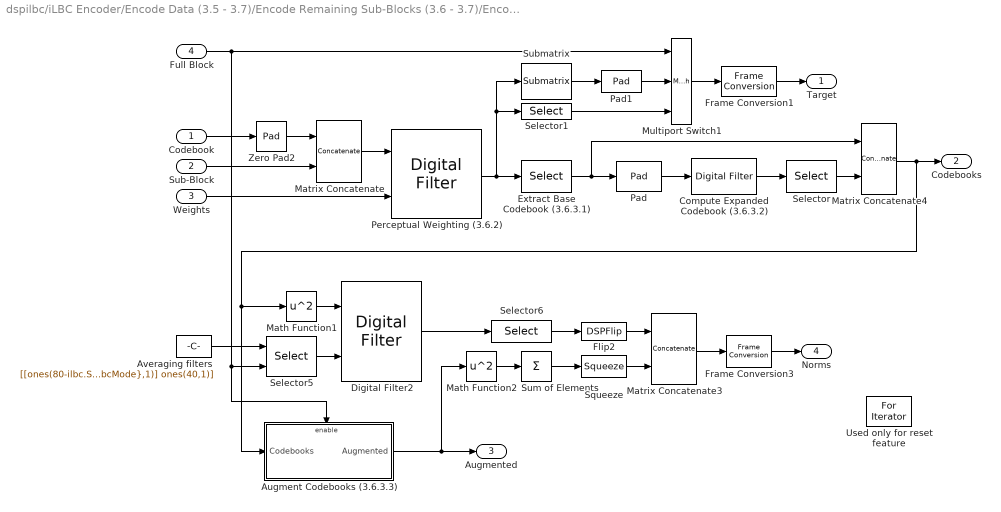
== system dspilbc/iLBC Encoder/Encode Data (3.5 - 3.7)/Encode Remaining Sub-Blocks (3.6 - 3.7)/Encode Sub-Block (3.6.2 - 3.7)/Compute Codebooks (3.6.2 - 3.6.3) ==
  Codebook : Inport
  Sub-Block : Inport  Port=2
  Weights : Inport  Port=3
  Full Block : Inport  Port=4
  Augment Codebooks (3.6.3.3) : Subsystem
  Averaging filters : Constant  Value=[[ones(80-ilbc.STATE_SHORT_LEN{ilbcMode},1); zeros(40-80+ilbc.STATE_SHORT_LEN{ilbcMode},1)] ones(40,1)]  OutDataTypeStr=Inherit: Inherit via back propagation
  Compute Expanded Codebook (3.6.3.2) : dsparch4/Digital Filter  TypePopup=FIR (all zeros)  IIRFiltStruct=Direct form II transposed  AllPoleFiltStruct=Direct form  FIRFiltStruct=Direct form  CoeffSource=Specify via dialog  NumCoeffs=ilbc.cbfiltersTbl  DenCoeffs=[-0.034180 0.108887 -0.184326 0.806152 0.713379 -0.144043 0.083740 -0.033691]  BiQuadCoeffs=[1 0.3 0.4 1 0.1 0.2]  LatticeCoeffs=[0.2 0.4]  denIgnore=on  FiltPerSampPopup=One filter per frame  IC=0  ICnum=0  ICden=0  roundingMode=Floor  overflowMode=off  ScaleValues=1  scaleValueFracLength=14  stageInFracLength=15  stageOutFracLength=15  FilterSource=Specify via dialog  dfiltObjectName=dfilt.dffir([1 2 1])  InputProcessing=Columns as channels (frame based)
  Digital Filter2 : dsparch4/Digital Filter  TypePopup=FIR (all zeros)  IIRFiltStruct=Direct form II transposed  AllPoleFiltStruct=Direct form  FIRFiltStruct=Direct form  CoeffSource=Input port(s)  NumCoeffs=[1 2]  DenCoeffs=[1 0.1]  BiQuadCoeffs=[1 0.3 0.4 1 0.1 0.2]  LatticeCoeffs=[0.2 0.4]  denIgnore=on  FiltPerSampPopup=One filter per frame  IC=0  ICnum=0  ICden=0  roundingMode=Floor  overflowMode=off  ScaleValues=1  scaleValueFracLength=14  stageInFracLength=15  stageOutFracLength=15  FilterSource=Input port(s)  dfiltObjectName=dfilt.dffir([1 2 1])  InputProcessing=Columns as channels (frame based)
  Extract Base Codebook (3.6.3.1) : Selector  NumberOfDimensions=2  InputPortWidth=151  IndexOptions=Index vector (dialog),Index vector (dialog)  Indices=1:147,1  OutputSizes=1,1
  Flip2 : DSPFlip
  Frame Conversion1 : FrameConversion  OutFrame=Sample-based
  Frame Conversion3 : FrameConversion  OutFrame=Sample-based
  Math Function1 : Math  Operator=square  SaturateOnIntegerOverflow=on
  Math Function2 : Math  Operator=square  SaturateOnIntegerOverflow=on
  Matrix Concatenate : Concatenate  Mode=Multidimensional array
  Matrix Concatenate3 : Concatenate  Mode=Multidimensional array
  Matrix Concatenate4 : Concatenate  Mode=Multidimensional array  ConcatenateDimension=2
  Multiport Switch1 : MultiPortSwitch  DataPortOrder=Zero-based contiguous  Inputs=2  zeroidx=on
  Pad : dspsigops/Pad  padAlong=Specified dimensions  dimsToPad=1  valSrc=Specify via dialog  padVal=0  spec=Pad size  padNumOutRowsSpecMethod=User-specified  numOutRows=1  padNumOutColsSpecMethod=User-specified  numOutCols=1  isVarDimsMode=off  padBeginning=0  padEnd=4  outSizeMode=User-specified  outSize=1  padSigAt=End  trunc_flag=None  roundingMode=Floor  overflowMode=off  truncOrWrapMode=Truncate  wrap_flag=None
  Pad1 : dspsigops/Pad  padAlong=Columns  dimsToPad=1  valSrc=Specify via dialog  padVal=0  spec=Output size  padNumOutRowsSpecMethod=User-specified  numOutRows=40  padNumOutColsSpecMethod=User-specified  numOutCols=1  isVarDimsMode=off  padBeginning=0  padEnd=0  outSizeMode=User-specified  outSize=1  padSigAt=Beginning  trunc_flag=None  roundingMode=Floor  overflowMode=off  truncOrWrapMode=Truncate  wrap_flag=None
  Perceptual Weighting (3.6.2) : dsparch4/Digital Filter  TypePopup=IIR (all poles)  IIRFiltStruct=Direct form II transposed  AllPoleFiltStruct=Direct form  FIRFiltStruct=Direct form  CoeffSource=Input port(s)  NumCoeffs=[1 2]  DenCoeffs=[1 0.1]  BiQuadCoeffs=[1 0.3 0.4 1 0.1 0.2]  LatticeCoeffs=[0.2 0.4]  denIgnore=off  FiltPerSampPopup=One filter per frame  IC=0  ICnum=0  ICden=0  roundingMode=Floor  overflowMode=off  ScaleValues=1  scaleValueFracLength=14  stageInFracLength=15  stageOutFracLength=15  FilterSource=Input port(s)  dfiltObjectName=dfilt.dffir([1 2 1])  InputProcessing=Columns as channels (frame based)
  Selector : Selector  NumberOfDimensions=2  InputPortWidth=151  IndexOptions=Index vector (dialog),Index vector (dialog)  Indices=5:151,1  OutputSizes=1,1
  Selector1 : Selector  NumberOfDimensions=2  InputPortWidth=151  IndexOptions=Index vector (dialog),Index vector (dialog)  Indices=148:187,1  OutputSizes=1,1
  Selector5 : Selector  NumberOfDimensions=2  IndexMode=Zero-based  InputPortWidth=3  IndexOptions=Select all,Index vector (port)  Indices=[1 3],1  OutputSizes=1,1
  Selector6 : Selector  NumberOfDimensions=2  InputPortWidth=3  IndexOptions=Index vector (dialog),Select all  Indices=40:147,1  OutputSizes=1,1
  Squeeze : Squeeze
  Submatrix : dspmtrx3/Submatrix  RowSpan=Range of rows  RowStartMode=Index  RowStartIndex=148  RowEndMode=Index  RowEndIndex=147+(80-ilbc.STATE_SHORT_LEN{ilbcMode})  ColSpan=All columns  ColStartMode=First  ColStartIndex=1  ColEndMode=Last  ColEndIndex=1
  Sum of Elements : Sum  Inputs=+  CollapseMode=Specified dimension  CollapseDim=2
  Used only for reset feature : ForIterator  ResetStates=reset  IterationLimit=1  ShowIterationPort=off
  Zero Pad2 : dspsigops/Pad  padAlong=Columns  dimsToPad=1  valSrc=Specify via dialog  padVal=0  spec=Output size  padNumOutRowsSpecMethod=User-specified  numOutRows=147  padNumOutColsSpecMethod=User-specified  numOutCols=1  isVarDimsMode=off  padBeginning=0  padEnd=0  outSizeMode=User-specified  outSize=1  padSigAt=Beginning  trunc_flag=None  roundingMode=Floor  overflowMode=off  truncOrWrapMode=Truncate  wrap_flag=None
  Target : Outport
  Codebooks : Outport  Port=2
  Augmented : Outport  Port=3
  Norms : Outport  Port=4
  wires:
  Selector/1 -> Matrix Concatenate4/2
  Squeeze/1 -> Matrix Concatenate3/2
  Augment Codebooks (3.6.3.3)/1(Augmented) -> Augmented/1, Math Function2/1
  Matrix Concatenate4/1 -> Math Function1/1, Augment Codebooks (3.6.3.3)/1(Codebooks), Codebooks/1
  Compute Expanded Codebook (3.6.3.2)/1 -> Selector/1
  Submatrix/1 -> Pad1/1
  Sum of Elements/1 -> Squeeze/1
  Math Function2/1 -> Sum of Elements/1
  Frame Conversion1/1 -> Target/1
  Frame Conversion3/1 -> Norms/1
  Full Block/1 -> Augment Codebooks (3.6.3.3)/Enable, Selector5/2, Multiport Switch1/1
  Perceptual Weighting (3.6.2)/1 -> Selector1/1, Submatrix/1, Extract Base Codebook (3.6.3.1)/1
  Extract Base Codebook (3.6.3.1)/1 -> Pad/1, Matrix Concatenate4/1
  Matrix Concatenate3/1 -> Frame Conversion3/1
  Math Function1/1 -> Digital Filter2/1
  Digital Filter2/1 -> Selector6/1
  Selector6/1 -> Flip2/1
  Selector5/1 -> Digital Filter2/2
  Averaging filters/1 -> Selector5/1
  Codebook/1 -> Zero Pad2/1
  Sub-Block/1 -> Matrix Concatenate/2
  Weights/1 -> Perceptual Weighting (3.6.2)/2
  Zero Pad2/1 -> Matrix Concatenate/1
  Matrix Concatenate/1 -> Perceptual Weighting (3.6.2)/1
  Pad/1 -> Compute Expanded Codebook (3.6.3.2)/1
  Flip2/1 -> Matrix Concatenate3/1
  Multiport Switch1/1 -> Frame Conversion1/1
  Pad1/1 -> Multiport Switch1/2
  Selector1/1 -> Multiport Switch1/3

== system dspilbc/iLBC Encoder/Encode Data (3.5 - 3.7)/Extract Sub-Blocks (3.5.1) and Sort LPC Filters/Parse Blocks/Flip Full Blocks ==
  Sub-blocks : Inport
  Start State Number : Inport  Port=2
  Assignment : Assignment  NumberOfDimensions=2  IndexMode=Zero-based  OutputInitialize=Specify size for each dimension in table  IndexOptions=Assign all,Index vector (port)  Indices=-1,1  OutputSizes=40,ilbc.NSUB{ilbcMode}-2
  Constant : Constant  Value=ilbc.NSUB{ilbcMode}-2  OutDataTypeStr=Inherit: Inherit via back propagation
  Flip1 : DSPFlip
  For Iterator : ForIterator  IterationLimit=ilbc.NSUB{ilbcMode}-2  IndexMode=Zero-based
  Multiport Switch2 : MultiPortSwitch  DataPortOrder=Zero-based contiguous  Inputs=2  zeroidx=on
  Relational Operator : RelationalOperator  OutDataTypeStr=boolean
  Selector1 : Selector  NumberOfDimensions=2  IndexMode=Zero-based  InputPortWidth=3  IndexOptions=Select all,Index vector (port)  Indices=-1,-1
  Sum : Sum  Inputs=+-|
  Flipped : Outport
  wires:
  For Iterator/1 -> Assignment/2, Selector1/2, Sum/2
  Constant/1 -> Sum/1
  Start State Number/1 -> Relational Operator/2
  Sum/1 -> Relational Operator/1
  Relational Operator/1 -> Multiport Switch2/1
  Flip1/1 -> Multiport Switch2/2
  Assignment/1 -> Flipped/1
  Multiport Switch2/1 -> Assignment/1
  Selector1/1 -> Multiport Switch2/3, Flip1/1
  Sub-blocks/1 -> Selector1/1

== system dspilbc/iLBC Encoder/Encode Data (3.5 - 3.7)/Encode Remaining Sub-Blocks (3.6 - 3.7)/Encode Sub-Block (3.6.2 - 3.7)/3 Stage Sub-Block Encoder (3.6.4)/Compute Correlations (3.6.4.1) ==
  Codebooks : Inport
  Augmented : Inport  Port=2
  Target : Inport  Port=3
  Array-Vector Multiply : dspmtrx3/Array-Vector Multiply  mode=Mute  saveAsFlag=0  Dimension=2  V_Source=Input port  V_VectFromMask=[0.5 0.25]  firstCoeffSignedness=Auto  firstCoeffDataTypeStr=Inherit: Same word length as input  firstCoeffLastDataTypeStr=Inherit: Same word length as input  firstCoeffMin=[]  firstCoeffMax=[]  outputSignedness=Auto  outputDataTypeStr=Inherit: Same as product output  outputLastDataTypeStr=Inherit: Same as product output  outputMin=[]  outputMax=[]  accumSignedness=Auto  prodOutputSignedness=Auto  roundingMode=Floor  overflowMode=off
  Digital Filter : dsparch4/Digital Filter  TypePopup=FIR (all zeros)  IIRFiltStruct=Direct form II transposed  AllPoleFiltStruct=Direct form  FIRFiltStruct=Direct form  CoeffSource=Input port(s)  NumCoeffs=[1 2]  DenCoeffs=[1 0.1]  BiQuadCoeffs=[1 0.3 0.4 1 0.1 0.2]  LatticeCoeffs=[0.2 0.4]  denIgnore=on  FiltPerSampPopup=One filter per frame  IC=0  ICnum=0  ICden=0  roundingMode=Floor  overflowMode=off  ScaleValues=1  scaleValueFracLength=14  stageInFracLength=15  stageOutFracLength=15  FilterSource=Input port(s)  dfiltObjectName=dfilt.dffir([1 2 1])  InputProcessing=Columns as channels (frame based)
  Flip : DSPFlip
  Flip1 : DSPFlip
  Frame Conversion2 : FrameConversion  OutFrame=Sample-based
  Matrix Concatenate1 : Concatenate  Mode=Multidimensional array
  Squeeze : Squeeze
  Submatrix : dspmtrx3/Submatrix  RowSpan=Range of rows  RowStartMode=Offset from last  RowStartIndex=107  RowEndMode=Last  RowEndIndex=1  ColSpan=All columns  ColStartMode=First  ColStartIndex=1  ColEndMode=Last  ColEndIndex=1
  Sum of Elements : Sum  Inputs=+  CollapseMode=Specified dimension  CollapseDim=2
  Correlations : Outport
  wires:
  Squeeze/1 -> Matrix Concatenate1/2
  Array-Vector Multiply/1 -> Sum of Elements/1
  Frame Conversion2/1 -> Correlations/1
  Flip/1 -> Digital Filter/2
  Submatrix/1 -> Flip1/1
  Flip1/1 -> Matrix Concatenate1/1
  Digital Filter/1 -> Submatrix/1
  Augmented/1 -> Array-Vector Multiply/1
  Codebooks/1 -> Digital Filter/1
  Sum of Elements/1 -> Squeeze/1
  Matrix Concatenate1/1 -> Frame Conversion2/1
  Target/1 -> Array-Vector Multiply/2, Flip/1

== system dspilbc/iLBC Encoder/Encode Data (3.5 - 3.7)/Encode Remaining Sub-Blocks (3.6 - 3.7)/Encode Sub-Block (3.6.2 - 3.7)/3 Stage Sub-Block Encoder (3.6.4)/Encode Gain (3.6.4.2) ==
  Stage : Inport
  Gain Value : Inport  Port=2
  Last Quantized Gain : Inport  Port=3
  Abs : Abs  OutDataTypeStr=Inherit: Inherit via back propagation
  Constant1 : Constant  Value=[ilbc.gain_sq5Tbl; ilbc.gain_sq4Tbl; ilbc.gain_sq3Tbl]  VectorParams1D=off  OutDataTypeStr=Inherit: Inherit via back propagation
  Data Type Duplicate1 : DataTypeDuplicate
  Product : Product  OutDataTypeStr=Inherit: Inherit via back propagation  RndMeth=Zero
  Saturation1 : Saturate  UpperLimit=inf  LowerLimit=0.1  OutDataTypeStr=Inherit: Inherit via back propagation
  Selector1 : Selector  NumberOfDimensions=2  IndexMode=Zero-based  InputPortWidth=3  IndexOptions=Index vector (port),Select all  Indices=1,1  OutputSizes=1,1
  VQ Encoder : dspquant2/Vector Quantizer Encoder  CBsource=Input port  codebook=GainCBs{Iteration}  distMeasure=Squared error  wgtSrc=Specify via dialog  weights=[1 1 1]  tieBreakRule=Choose the lower index  outQU=on  outQError=off  idtype=uint8  roundingMode=Floor  overflowMode=off
  Gain Index : Outport
  Quantized Gain : Outport  Port=2
  wires:
  Stage/1 -> Selector1/2
  Constant1/1 -> Data Type Duplicate1/2, Selector1/1
  Selector1/1 -> Product/1
  Gain Value/1 -> VQ Encoder/1
  VQ Encoder/2 -> Quantized Gain/1
  VQ Encoder/1 -> Gain Index/1
  Product/1 -> VQ Encoder/2
  Abs/1 -> Saturation1/1
  Saturation1/1 -> Product/2
  Last Quantized Gain/1 -> Data Type Duplicate1/1, Abs/1
